simulink model "RCAMVisualization_Model"  (R2021a)
settings: Solver=ode45  StartTime=0.0  StopTime=simulation.t_final  RelTol=1e-3  EnableMultiTasking=on
libraries: UWAerospaceBlockset_EquationsOfMotion x4, aerolibfltsims x2, UWAerospaceBlockset_Animation x2, aerolibanimutils x1
settings Model: Creator=lum  LastModifiedBy=chris
settings SolverCC: AlgebraicLoopSolver=TrustRegion
settings DataIOCC: LimitDataPoints=on  SaveFormat=Array  ReturnWorkspaceOutputs=off
settings OptimizationCC: ExpressionDepthLimit=2147483647  LifeSpan=inf
settings DebuggingCC: UnderspecifiedInitializationDetection=Classic  MergeDetectMultiDrivingBlocksExec=none  SolverPrmCheckMsg=warning  FcnCallInpInsideContextMsg=warning  StateNameClashWarn=warning  SFUnexpectedBacktrackingDiag=warning  SFNoUnconditionalDefaultTransitionDiag=warning  SFExecutionAtInitializationDiag=none  SFMachineParentedDataDiag=warning  ArithmeticOperatorsInVariantConditions=warning
settings HardwareCC: ProdBitPerPointer=32  ProdBitPerSizeT=32  ProdBitPerPtrDiffT=32  ProdLargestAtomicFloat=None  ProdIntDivRoundTo=Undefined  ProdEndianess=Unspecified  ProdWordSize=32  ProdHWDeviceType=32-bit Generic
settings ModelReferenceCC: PropagateSignalLabelsOutOfModel=off
settings SFSimCC: SimUseLocalCustomCode=off  CustomCodeUndefinedFunction=UseInterfaceOnly
settings RTWCC: RTWUseLocalCustomCode=off
settings CodeAppCC: StateflowObjectComments=on
settings GRTTargetCC: TargetLangStandard=C89/C90 (ANSI)  CombineOutputUpdateFcns=off  GRTInterface=on
settings ConfigComp: CovMetricSettings=dw  CovSaveCumulativeToWorkspaceVar=on  CovSaveSingleToWorkspaceVar=on  CovExternalEMLEnable=off  CovSFcnEnable=off

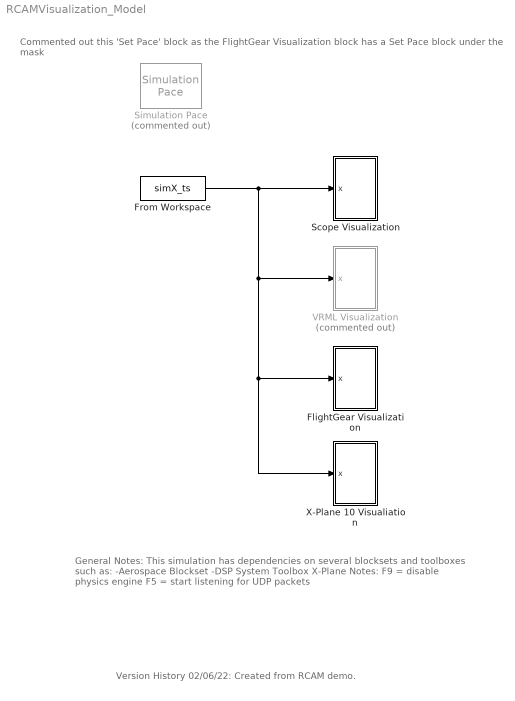
== system RCAMVisualization_Model ==
  note: Commented out this 'Set Pace' block as the FlightGear Visualization block has a Set Pace block under the mask
  note: General Notes:
      | This simulation has dependencies on several blocksets and toolboxes such as:
      | -Aerospace Blockset
      | -DSP System Toolbox
      |
      | X-Plane Notes:
      | F9 = disable physics engine
      | F5 = start listening for UDP packets
  note: Version History
      | 02/06/22: Created from RCAM demo.
  FlightGear Visualization : Subsystem
  From Workspace : FromWorkspace  VariableName=simX_ts
  Scope Visualization : Subsystem
  Simulation Pace : aerolibanimutils/Simulation Pace  Commented=on  SimulationPace=1  SleepMode=Auto  OutputPaceError=off  SampleTime=1/30
  VRML Visualization : Subsystem  Commented=on
  X-Plane 10 Visualiation : Subsystem
  wires:
  From Workspace/1 -> Scope Visualization/1(x), X-Plane 10 Visualiation/1(x), FlightGear Visualization/1(x), VRML Visualization/1(x)

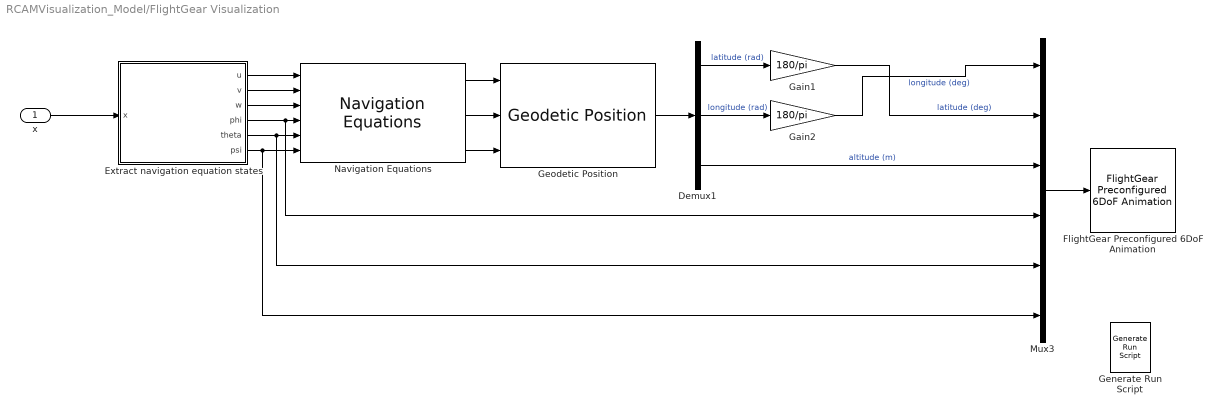
== system RCAMVisualization_Model/FlightGear Visualization ==
  x : Inport
  Demux1 : Demux  Outputs=3
  Extract navigation equation states : Subsystem
  FlightGear Preconfigured 6DoF Animation : aerolibfltsims/FlightGear Preconfigured 6DoF Animation  xFlightGearVersion=v2018.1  DestinationIpAddress=127.0.0.1  DestinationPort=5502  SampleTime=1/30  packetVersion=24
  Gain1 : Gain  Gain=180/pi
  Gain2 : Gain  Gain=180/pi
  Generate Run Script : aerolibfltsims/Generate Run Script  Architecture=Win64  dataFlow=Send  GeometryModelName=c172p  AirportId=KSFO  RunwayId=10L  InitialAltitude=7224  InitialHeading=113  OffsetDistance=4.72  OffsetAzimuth=0  InstallScenery=off  DisableShaders=on  OriginAddress=127.0.0.1  DestinationPort=5502  OriginPort=5505  LocalAddress=127.0.0.1  OutputFileName=runfg.bat  FlightGearBaseDirectory=C:\Program Files\FlightGear 2018.1.1
  Geodetic Position : UWAerospaceBlockset_EquationsOfMotion/Geodetic Position  Xgeodetic0=Xgeodetic0
  Mux3 : Mux  Inputs=6
  Navigation Equations : UWAerospaceBlockset_EquationsOfMotion/Navigation Equations  Description=|
      | Version History  
      |                  
      | 05/24/05: Created
  wires:
  Demux1/3 -> Mux3/3  "altitude (m)"
  Gain1/1 -> Mux3/2  "latitude (deg)"
  Demux1/1 -> Gain1/1  "latitude (rad)"
  Navigation Equations/1 -> Geodetic Position/1
  Navigation Equations/3 -> Geodetic Position/3
  Demux1/2 -> Gain2/1  "longitude (rad)"
  Extract navigation equation states/4(phi) -> Mux3/4, Navigation Equations/4
  Extract navigation equation states/6(psi) -> Mux3/6, Navigation Equations/6
  Extract navigation equation states/1(u) -> Navigation Equations/1
  Navigation Equations/2 -> Geodetic Position/2
  Gain2/1 -> Mux3/1  "longitude (deg)"
  Extract navigation equation states/5(theta) -> Mux3/5, Navigation Equations/5
  Extract navigation equation states/2(v) -> Navigation Equations/2
  Extract navigation equation states/3(w) -> Navigation Equations/3
  Mux3/1 -> FlightGear Preconfigured 6DoF Animation/1
  Geodetic Position/1 -> Demux1/1
  x/1 -> Extract navigation equation states/1(x)

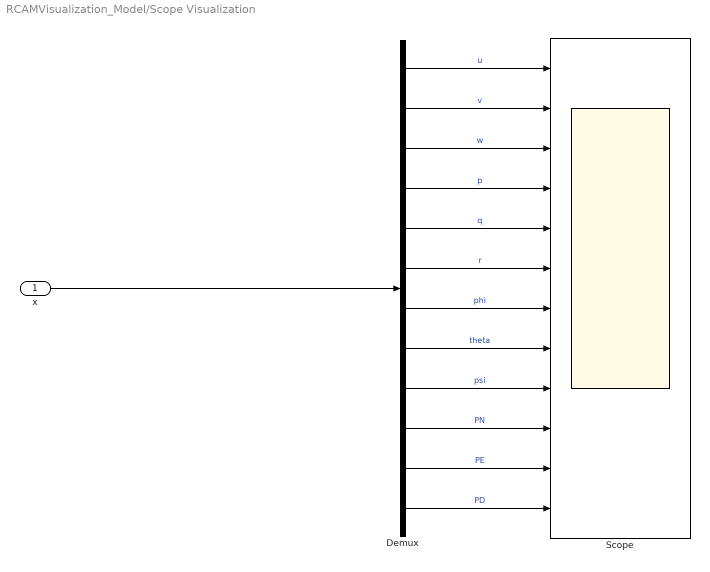
== system RCAMVisualization_Model/Scope Visualization ==
  x : Inport
  Demux : Demux  Outputs=12
  Scope : Scope  NumInputPorts=12
  wires:
  x/1 -> Demux/1
  Demux/3 -> Scope/3  "w"
  Demux/2 -> Scope/2  "v"
  Demux/4 -> Scope/4  "p"
  Demux/1 -> Scope/1  "u"
  Demux/5 -> Scope/5  "q"
  Demux/6 -> Scope/6  "r"
  Demux/7 -> Scope/7  "phi"
  Demux/8 -> Scope/8  "theta"
  Demux/9 -> Scope/9  "psi"
  Demux/10 -> Scope/10  "PN"
  Demux/11 -> Scope/11  "PE"
  Demux/12 -> Scope/12  "PD"

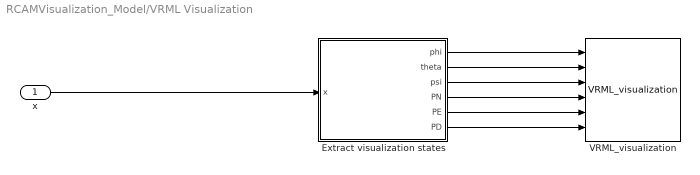
== system RCAMVisualization_Model/VRML Visualization ==
  x : Inport
  Extract visualization states : Subsystem
  VRML_visualization : UWAerospaceBlockset_Animation/VRML_visualization
  wires:
  Extract visualization states/2(theta) -> VRML_visualization/2
  Extract visualization states/1(phi) -> VRML_visualization/1
  Extract visualization states/5(PE) -> VRML_visualization/5
  Extract visualization states/6(PD) -> VRML_visualization/6
  Extract visualization states/4(PN) -> VRML_visualization/4
  Extract visualization states/3(psi) -> VRML_visualization/3
  x/1 -> Extract visualization states/1(x)

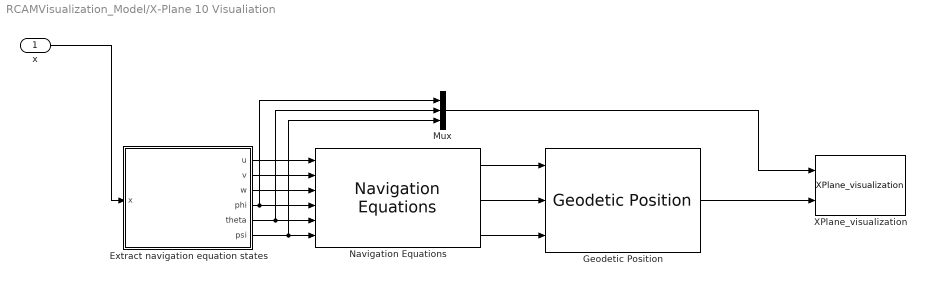
== system RCAMVisualization_Model/X-Plane 10 Visualiation ==
  x : Inport
  Extract navigation equation states : Subsystem
  Geodetic Position : UWAerospaceBlockset_EquationsOfMotion/Geodetic Position  Xgeodetic0=Xgeodetic0
  Mux : Mux  Inputs=3
  Navigation Equations : UWAerospaceBlockset_EquationsOfMotion/Navigation Equations  Description=|
      | Version History  
      |                  
      | 05/24/05: Created
  XPlane_visualization : UWAerospaceBlockset_Animation/XPlane_visualization  IP_address=simulation.x_plane.state_visualization.IP_address  plugin_listening_port_number=simulation.x_plane.state_visualization.plugin_listening_port_number  numDigitsOfPrecision=simulation.x_plane.state_visualization.numDigitsOfPrecision
  wires:
  Navigation Equations/2 -> Geodetic Position/2
  Geodetic Position/1 -> XPlane_visualization/2
  Extract navigation equation states/2(v) -> Navigation Equations/2
  Extract navigation equation states/4(phi) -> Mux/1, Navigation Equations/4
  Extract navigation equation states/1(u) -> Navigation Equations/1
  Navigation Equations/1 -> Geodetic Position/1
  x/1 -> Extract navigation equation states/1(x)
  Extract navigation equation states/6(psi) -> Mux/3, Navigation Equations/6
  Navigation Equations/3 -> Geodetic Position/3
  Extract navigation equation states/3(w) -> Navigation Equations/3
  Extract navigation equation states/5(theta) -> Mux/2, Navigation Equations/5
  Mux/1 -> XPlane_visualization/1

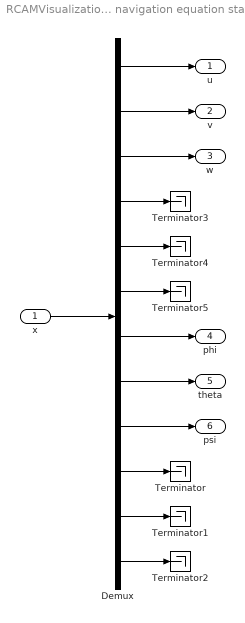
== system RCAMVisualization_Model/FlightGear Visualization/Extract navigation equation states ==
  x : Inport
  Demux : Demux  Outputs=12
  Terminator{,1..5} (6 alike) : Terminator
  u : Outport  VectorParamsAs1DForOutWhenUnconnected=off
  v : Outport  Port=2  VectorParamsAs1DForOutWhenUnconnected=off
  w : Outport  Port=3  VectorParamsAs1DForOutWhenUnconnected=off
  phi : Outport  Port=4  VectorParamsAs1DForOutWhenUnconnected=off
  theta : Outport  Port=5  VectorParamsAs1DForOutWhenUnconnected=off
  psi : Outport  Port=6  VectorParamsAs1DForOutWhenUnconnected=off
  wires:
  Demux/6 -> Terminator5/1
  Demux/5 -> Terminator4/1
  Demux/4 -> Terminator3/1
  x/1 -> Demux/1
  Demux/1 -> u/1
  Demux/2 -> v/1
  Demux/3 -> w/1
  Demux/7 -> phi/1
  Demux/8 -> theta/1
  Demux/9 -> psi/1
  Demux/10 -> Terminator/1
  Demux/11 -> Terminator1/1
  Demux/12 -> Terminator2/1

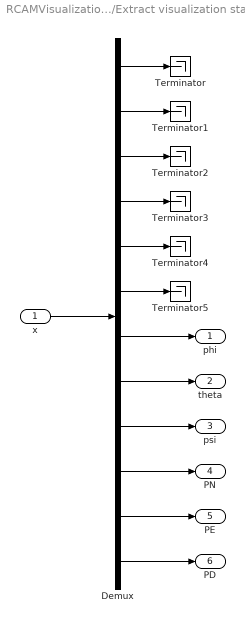
== system RCAMVisualization_Model/VRML Visualization/Extract visualization states ==
  x : Inport
  Demux : Demux  Outputs=12
  Terminator{,1..5} (6 alike) : Terminator
  phi : Outport  VectorParamsAs1DForOutWhenUnconnected=off
  theta : Outport  Port=2  VectorParamsAs1DForOutWhenUnconnected=off
  psi : Outport  Port=3  VectorParamsAs1DForOutWhenUnconnected=off
  PN : Outport  Port=4  VectorParamsAs1DForOutWhenUnconnected=off
  PE : Outport  Port=5  VectorParamsAs1DForOutWhenUnconnected=off
  PD : Outport  Port=6  VectorParamsAs1DForOutWhenUnconnected=off
  wires:
  x/1 -> Demux/1
  Demux/1 -> Terminator/1
  Demux/2 -> Terminator1/1
  Demux/3 -> Terminator2/1
  Demux/4 -> Terminator3/1
  Demux/5 -> Terminator4/1
  Demux/6 -> Terminator5/1
  Demux/7 -> phi/1
  Demux/8 -> theta/1
  Demux/9 -> psi/1
  Demux/10 -> PN/1
  Demux/11 -> PE/1
  Demux/12 -> PD/1

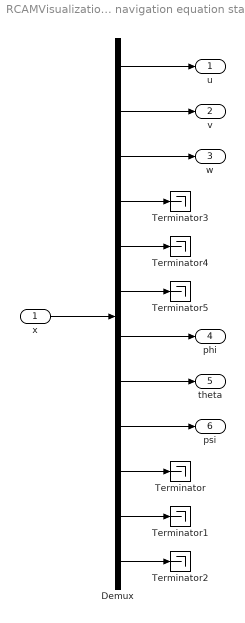
== system RCAMVisualization_Model/X-Plane 10 Visualiation/Extract navigation equation states ==
  x : Inport
  Demux : Demux  Outputs=12
  Terminator{,1..5} (6 alike) : Terminator
  u : Outport  VectorParamsAs1DForOutWhenUnconnected=off
  v : Outport  Port=2  VectorParamsAs1DForOutWhenUnconnected=off
  w : Outport  Port=3  VectorParamsAs1DForOutWhenUnconnected=off
  phi : Outport  Port=4  VectorParamsAs1DForOutWhenUnconnected=off
  theta : Outport  Port=5  VectorParamsAs1DForOutWhenUnconnected=off
  psi : Outport  Port=6  VectorParamsAs1DForOutWhenUnconnected=off
  wires:
  Demux/6 -> Terminator5/1
  Demux/5 -> Terminator4/1
  Demux/4 -> Terminator3/1
  x/1 -> Demux/1
  Demux/1 -> u/1
  Demux/2 -> v/1
  Demux/3 -> w/1
  Demux/7 -> phi/1
  Demux/8 -> theta/1
  Demux/9 -> psi/1
  Demux/10 -> Terminator/1
  Demux/11 -> Terminator1/1
  Demux/12 -> Terminator2/1
